simulink model "CoETS"  (R2018a)
settings: configuration reference "cs_ert" (kept outside this file)
settings Model: DataDictionary=CoETS.sldd  Creator=zhoutinglin  LastModifiedBy=zhoutinglin

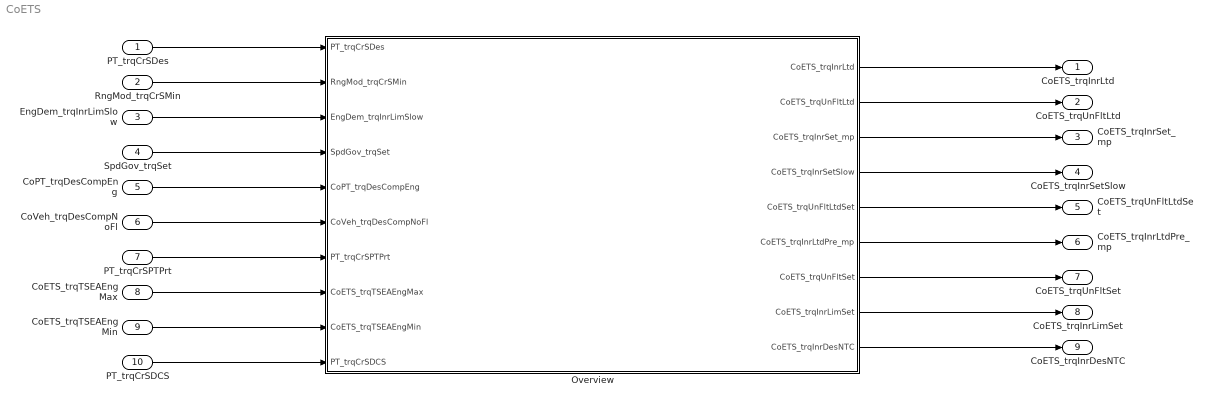
== system CoETS ==
  PT_trqCrSDes : Inport
  RngMod_trqCrSMin : Inport  Port=2
  EngDem_trqInrLimSlow : Inport  Port=3
  SpdGov_trqSet : Inport  Port=4
  CoPT_trqDesCompEng : Inport  Port=5
  CoVeh_trqDesCompNoFl : Inport  Port=6
  PT_trqCrSPTPrt : Inport  Port=7
  CoETS_trqTSEAEngMax : Inport  Port=8
  CoETS_trqTSEAEngMin : Inport  Port=9
  PT_trqCrSDCS : Inport  Port=10
  Overview : Subsystem
  CoETS_trqInrLtd : Outport
  CoETS_trqUnFltLtd : Outport  Port=2
  CoETS_trqInrSet_mp : Outport  Port=3
  CoETS_trqInrSetSlow : Outport  Port=4
  CoETS_trqUnFltLtdSet : Outport  Port=5
  CoETS_trqInrLtdPre_mp : Outport  Port=6
  CoETS_trqUnFltSet : Outport  Port=7
  CoETS_trqInrLimSet : Outport  Port=8
  CoETS_trqInrDesNTC : Outport  Port=9
  wires:
  PT_trqCrSDes/1 -> Overview/1(PT_trqCrSDes)
  RngMod_trqCrSMin/1 -> Overview/2(RngMod_trqCrSMin)
  EngDem_trqInrLimSlow/1 -> Overview/3(EngDem_trqInrLimSlow)
  SpdGov_trqSet/1 -> Overview/4(SpdGov_trqSet)
  CoPT_trqDesCompEng/1 -> Overview/5(CoPT_trqDesCompEng)
  CoVeh_trqDesCompNoFl/1 -> Overview/6(CoVeh_trqDesCompNoFl)
  PT_trqCrSPTPrt/1 -> Overview/7(PT_trqCrSPTPrt)
  CoETS_trqTSEAEngMax/1 -> Overview/8(CoETS_trqTSEAEngMax)
  CoETS_trqTSEAEngMin/1 -> Overview/9(CoETS_trqTSEAEngMin)
  PT_trqCrSDCS/1 -> Overview/10(PT_trqCrSDCS)
  Overview/1(CoETS_trqInrLtd) -> CoETS_trqInrLtd/1
  Overview/2(CoETS_trqUnFltLtd) -> CoETS_trqUnFltLtd/1
  Overview/3(CoETS_trqInrSet_mp) -> CoETS_trqInrSet_mp/1
  Overview/4(CoETS_trqInrSetSlow) -> CoETS_trqInrSetSlow/1
  Overview/5(CoETS_trqUnFltLtdSet) -> CoETS_trqUnFltLtdSet/1
  Overview/6(CoETS_trqInrLtdPre_mp) -> CoETS_trqInrLtdPre_mp/1
  Overview/7(CoETS_trqUnFltSet) -> CoETS_trqUnFltSet/1
  Overview/8(CoETS_trqInrLimSet) -> CoETS_trqInrLimSet/1
  Overview/9(CoETS_trqInrDesNTC) -> CoETS_trqInrDesNTC/1

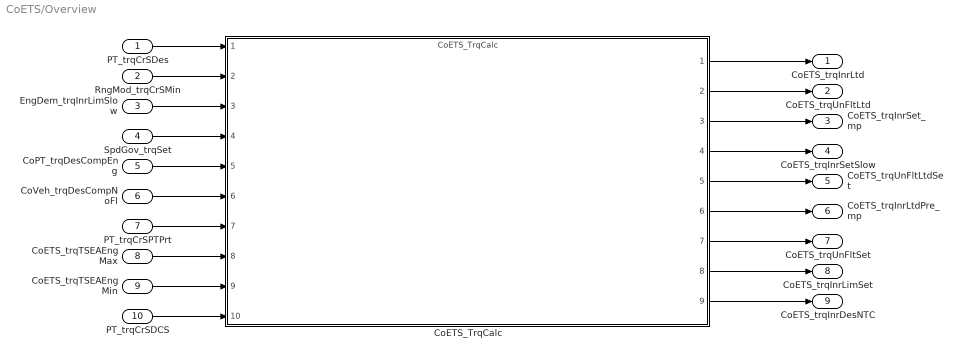
== system CoETS/Overview ==
  PT_trqCrSDes : Inport
  RngMod_trqCrSMin : Inport  Port=2
  EngDem_trqInrLimSlow : Inport  Port=3
  SpdGov_trqSet : Inport  Port=4
  CoPT_trqDesCompEng : Inport  Port=5
  CoVeh_trqDesCompNoFl : Inport  Port=6
  PT_trqCrSPTPrt : Inport  Port=7
  CoETS_trqTSEAEngMax : Inport  Port=8
  CoETS_trqTSEAEngMin : Inport  Port=9
  PT_trqCrSDCS : Inport  Port=10
  CoETS_TrqCalc : ModelReference  ModelNameDialog=CoETS_TrqCalc  SimulationMode=Normal  ModelReferenceVersion=1.54
  CoETS_trqInrLtd : Outport
  CoETS_trqUnFltLtd : Outport  Port=2
  CoETS_trqInrSet_mp : Outport  Port=3
  CoETS_trqInrSetSlow : Outport  Port=4
  CoETS_trqUnFltLtdSet : Outport  Port=5
  CoETS_trqInrLtdPre_mp : Outport  Port=6
  CoETS_trqUnFltSet : Outport  Port=7
  CoETS_trqInrLimSet : Outport  Port=8
  CoETS_trqInrDesNTC : Outport  Port=9
  wires:
  PT_trqCrSDes/1 -> CoETS_TrqCalc/1
  RngMod_trqCrSMin/1 -> CoETS_TrqCalc/2
  EngDem_trqInrLimSlow/1 -> CoETS_TrqCalc/3
  SpdGov_trqSet/1 -> CoETS_TrqCalc/4
  CoPT_trqDesCompEng/1 -> CoETS_TrqCalc/5
  CoVeh_trqDesCompNoFl/1 -> CoETS_TrqCalc/6
  PT_trqCrSPTPrt/1 -> CoETS_TrqCalc/7
  CoETS_trqTSEAEngMax/1 -> CoETS_TrqCalc/8
  CoETS_trqTSEAEngMin/1 -> CoETS_TrqCalc/9
  PT_trqCrSDCS/1 -> CoETS_TrqCalc/10
  CoETS_TrqCalc/1 -> CoETS_trqInrLtd/1
  CoETS_TrqCalc/2 -> CoETS_trqUnFltLtd/1
  CoETS_TrqCalc/3 -> CoETS_trqInrSet_mp/1
  CoETS_TrqCalc/4 -> CoETS_trqInrSetSlow/1
  CoETS_TrqCalc/5 -> CoETS_trqUnFltLtdSet/1
  CoETS_TrqCalc/6 -> CoETS_trqInrLtdPre_mp/1
  CoETS_TrqCalc/7 -> CoETS_trqUnFltSet/1
  CoETS_TrqCalc/8 -> CoETS_trqInrLimSet/1
  CoETS_TrqCalc/9 -> CoETS_trqInrDesNTC/1
